simulink model "L5_sim1"  (R2024b)
settings: Solver=VariableStepAuto  StartTime=0.0  StopTime=100  RelTol=1e-3
values from neighbouring files (symbols this model uses):
  eul_0 = [0, 0, 0]'    [Task1.m]    (also in Task2.m)
  I = diag([Ix, Iy, Iz])    [Task1.m]    (also in Task2.m)
  w_0 = [0.5, 0.0, 0.0]'    [Task1.m]    (also in Task2.m = [C, 0.1, 0.1]')
libraries: matrix_library x1
settings Model: Creator=alejandromunozvazquez  LastModifiedBy=alejandromunozvazquez

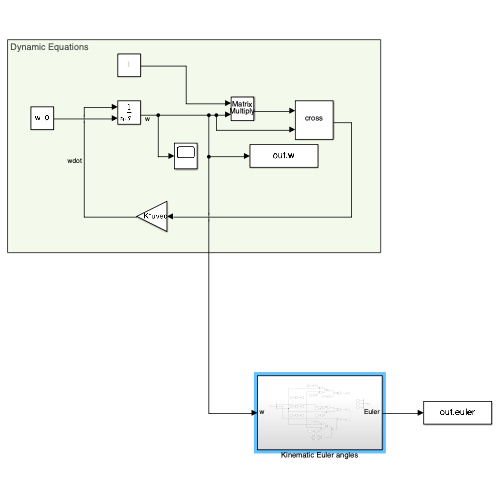
[thumbnail: Simulink's stored preview of the top-level diagram]
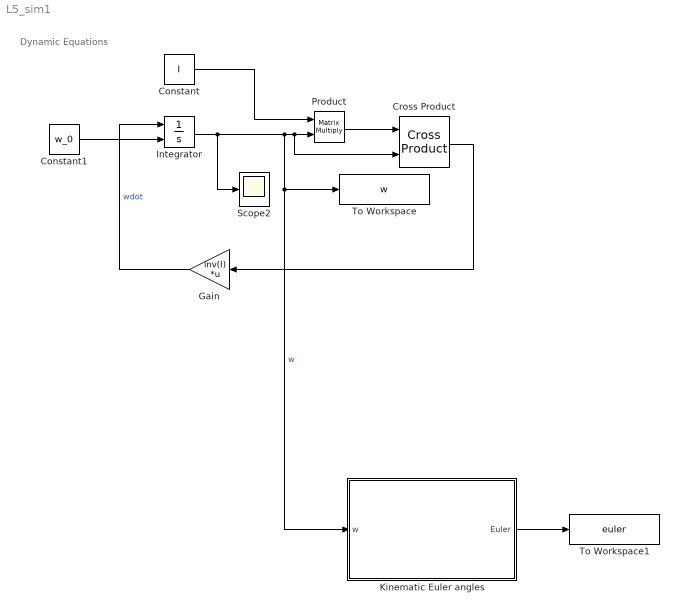
== system L5_sim1 ==
  note: Dynamic Equations
  Constant : Constant  Value=I
  Constant1 : Constant  Value=w_0
  Cross Product : matrix_library/Cross Product
  Gain : Gain  Gain=inv(I)  Multiplication=Matrix(K*u) (u vector)
  Integrator : Integrator  InitialConditionSource=external
  Kinematic Euler angles : Subsystem
  Product : Product  Multiplication=Matrix(*)
  Scope2 : Scope
  To Workspace : ToWorkspace  VariableName=w  SampleTime=-1
  To Workspace1 : ToWorkspace  VariableName=euler  SampleTime=-1
  wires:
  Gain/1 -> Integrator/1  "wdot"
  Integrator/1 -> Scope2/1, Product/2, Cross Product/2, Kinematic Euler angles/1(w), To Workspace/1  "w"
  Constant/1 -> Product/1
  Product/1 -> Cross Product/1
  Cross Product/1 -> Gain/1
  Constant1/1 -> Integrator/2
  Kinematic Euler angles/1(Euler) -> To Workspace1/1

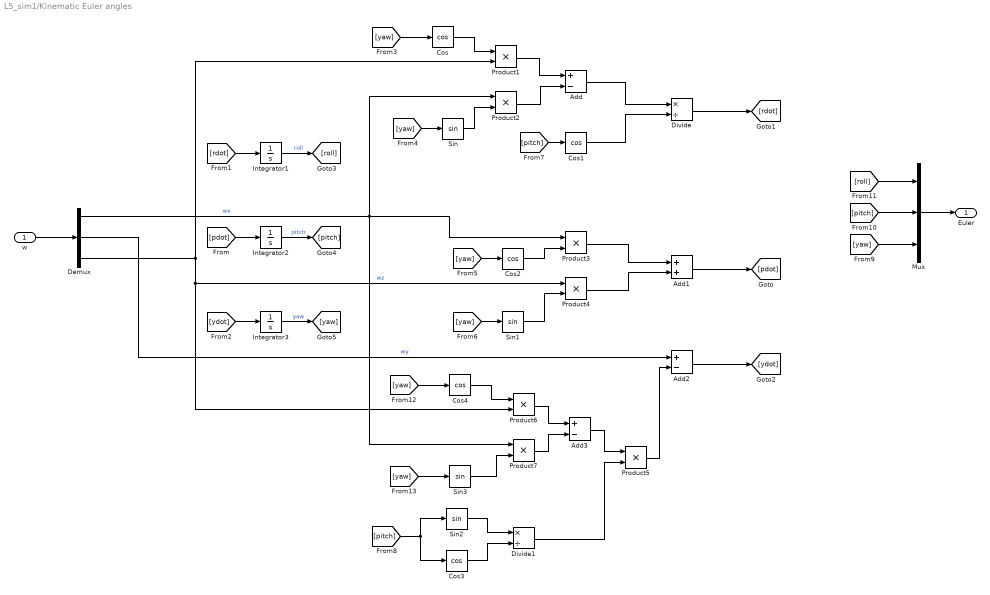
== system L5_sim1/Kinematic Euler angles ==
  w : Inport
  Add : Sum  Inputs=+-
  Add1 : Sum
  Add2 : Sum  Inputs=+-
  Add3 : Sum  Inputs=+-
  Cos{,1..4} (5 alike) : Trigonometry  Operator=cos
  Demux : Demux  Outputs=3
  Divide : Product  Inputs=*/
  Divide1 : Product  Inputs=*/
  Integrator1 : Integrator  InitialCondition=eul_0(1)
  Integrator2 : Integrator  InitialCondition=eul_0(2)
  Integrator3 : Integrator  InitialCondition=eul_0(3)
  Mux : Mux  Inputs=3
  Product{1..7} (7 alike) : Product
  Sin{,1..3} (4 alike) : Trigonometry
  Euler : Outport
  wires:
  w/1 -> Demux/1
  Sin1/1 -> Product4/2
  [ydot] -> Integrator3/1
  Sin/1 -> Product2/2
  Divide/1 -> [rdot]
  Cos/1 -> Product1/1
  Product3/1 -> Add1/1
  Demux/3 -> Product1/2, Product6/2, Product4/1  "wz"
  Product4/1 -> Add1/2
  Product1/1 -> Add/1
  Add/1 -> Divide/1
  Product2/1 -> Add/2
  Add1/1 -> [pdot]
  Sin2/1 -> Divide1/1
  Integrator2/1 -> [pitch]  "pitch"
  Cos3/1 -> Divide1/2
  [rdot] -> Integrator1/1
  Demux/1 -> Product3/1, Product2/1, Product7/1  "wx"
  Integrator1/1 -> [roll]  "roll"
  Add2/1 -> [ydot]
  [pdot] -> Integrator2/1
  Cos1/1 -> Divide/2
  Cos2/1 -> Product3/2
  Demux/2 -> Add2/1  "wy"
  Integrator3/1 -> [yaw]  "yaw"
  Mux/1 -> Euler/1
  [yaw] -> Cos/1
  [yaw] -> Sin/1
  [yaw] -> Cos2/1
  [yaw] -> Sin1/1
  [pitch] -> Cos1/1
  [pitch] -> Sin2/1, Cos3/1
  [yaw] -> Mux/3
  [pitch] -> Mux/2
  [roll] -> Mux/1
  Product5/1 -> Add2/2
  [yaw] -> Cos4/1
  Cos4/1 -> Product6/1
  [yaw] -> Sin3/1
  Sin3/1 -> Product7/2
  Product6/1 -> Add3/1
  Product7/1 -> Add3/2
  Add3/1 -> Product5/1
  Divide1/1 -> Product5/2
